simulink library "Robot_daVinci_Lib"  (R2025b)
settings: Solver=VariableStepAuto  StartTime=0.0  StopTime=10.0  RelTol=1e-3
settings Model: Creator=raissare  LastModifiedBy=guilhermepifferchristo
settings RTWCC: GPUComputeCapability=3.5

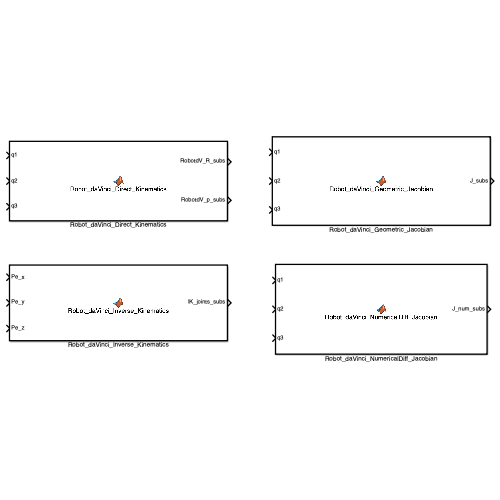
[thumbnail: Simulink's stored preview of the top-level diagram]
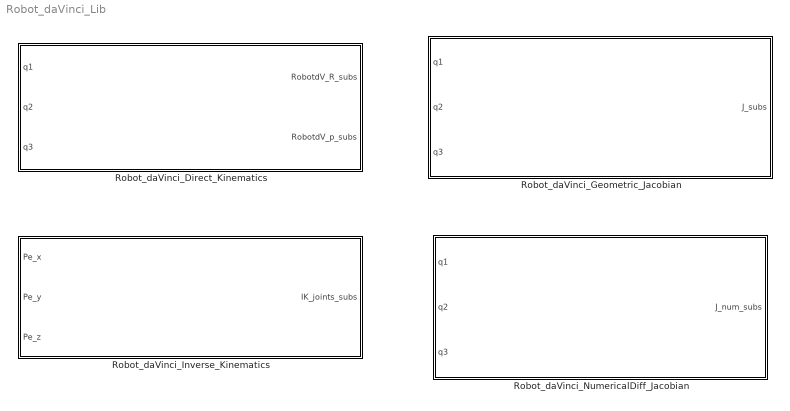
== system Robot_daVinci_Lib ==
  Robot_daVinci_Direct_Kinematics : MATLAB Function  TreatAsAtomicUnit=on
  Robot_daVinci_Geometric_Jacobian : MATLAB Function  TreatAsAtomicUnit=on
  Robot_daVinci_Inverse_Kinematics : MATLAB Function  TreatAsAtomicUnit=on
  Robot_daVinci_NumericalDiff_Jacobian : MATLAB Function  TreatAsAtomicUnit=on

== matlab function Robot_daVinci_Lib/Robot_daVinci_Geometric_Jacobian ==
  data: q1 input; J_subs output; q2 input; q3 input
function J_subs = Robot_daVinci_Geometric_Jacobian(q1,q2,q3)
%#codegen

%    This function was generated by the Symbolic Math Toolbox version 25.2.
%    10-May-2026 17:21:34

% q1 = complex(q1);  % if required to enforce complex operations
% q2 = complex(q2);  % if required to enforce complex operations
% q3 = complex(q3);  % if required to enforce complex operations
t2 = cos(q1);
t3 = cos(q2);
t4 = sin(q1);
t5 = sin(q2);
t6 = q3.*t3;
t7 = q3.*t2.*t5;
t8 = q3.*t4.*t5;
t10 = t5./1.0e+1;
t11 = (t2.*t3)./1.0e+1;
t12 = (t3.*t4)./1.0e+1;
t9 = -t6;
t14 = t7+t11;
t13 = t9+t10;
J_subs = reshape([-t8-t12,t14,0.0,0.0,0.0,1.0,-t2.*t13,-t4.*t13,t4.*(t8+t12)+t2.*t14,t4,-t2,0.0,t2.*t5,t4.*t5,-t3,0.0,0.0,0.0],[6,3]);
end

== matlab function Robot_daVinci_Lib/Robot_daVinci_Direct_Kinematics ==
  data: q1 input; RobotdV_R_subs output; q2 input; q3 input; RobotdV_p_subs output
function [RobotdV_R_subs,RobotdV_p_subs] = Robot_daVinci_Direct_Kinematics(q1,q2,q3)
%#codegen

%    This function was generated by the Symbolic Math Toolbox version 25.2.
%    10-May-2026 17:21:32

% q1 = complex(q1);  % if required to enforce complex operations
% q2 = complex(q2);  % if required to enforce complex operations
% q3 = complex(q3);  % if required to enforce complex operations
t2 = cos(q1);
t3 = cos(q2);
t4 = sin(q1);
t5 = sin(q2);
RobotdV_R_subs = reshape([t2.*t3,t3.*t4,t5,t4,-t2,0.0,t2.*t5,t4.*t5,-t3],[3,3]);
if nargout > 1
    t6 = q3.*t5;
    t7 = t3./1.0e+1;
    t8 = t6+t7;
    RobotdV_p_subs = [t2.*t8;t4.*t8;t5./1.0e+1-q3.*t3];
end
end

== matlab function Robot_daVinci_Lib/Robot_daVinci_NumericalDiff_Jacobian ==
  data: q1 input; J_num_subs output; q2 input; q3 input
function J_num_subs = Robot_daVinci_NumericalDiff_Jacobian(q1,q2,q3)
%#codegen

%    This function was generated by the Symbolic Math Toolbox version 25.2.
%    10-May-2026 17:21:34

% q1 = complex(q1);  % if required to enforce complex operations
% q2 = complex(q2);  % if required to enforce complex operations
% q3 = complex(q3);  % if required to enforce complex operations
t2 = cos(q1);
t3 = cos(q2);
t4 = sin(q1);
t5 = sin(q2);
t10 = q1+1.0e-6;
t11 = q2+1.0e-6;
t6 = t3.^2;
t7 = t5.^2;
t8 = q3.*t5;
t9 = t3./1.0e+1;
t12 = t2.*t4.*1.0e+6;
t13 = cos(t10);
t14 = cos(t11);
t15 = sin(t10);
t16 = sin(t11);
t20 = t3.*1.00001e-1;
t17 = t8+t9;
t18 = -t12;
t19 = q3.*t16;
t21 = t14./1.0e+1;
t22 = t8+t20;
t23 = t2.*t17.*1.0e+6;
t24 = t4.*t17.*1.0e+6;
t27 = t19+t21;
t25 = -t23;
t26 = -t24;
mt1 = [t25+t2.*t22.*1.0e+6,t26+t4.*t22.*1.0e+6,t5,0.0,0.0,t18+t6.*t12+t7.*t12,t25+t13.*t17.*1.0e+6,t26+t15.*t17.*1.0e+6,0.0,0.0,0.0,t4.*t13.*-1.0e+6+t2.*t6.*t15.*1.0e+6+t2.*t7.*t15.*1.0e+6,t25+t2.*t27.*1.0e+6,t26+t4.*t27.*1.0e+6,t5.*-1.0e+5+t16.*1.0e+5+q3.*t3.*1.0e+6-q3.*t14.*1.0e+6,t3.*t4.*t16.*1.0e+6-t4.*t5.*t14.*1.0e+6];
mt2 = [t2.*t3.*t16.*-1.0e+6+t2.*t5.*t14.*1.0e+6,t18+t3.*t12.*t14+t5.*t12.*t16];
J_num_subs = reshape([mt1,mt2],6,3);
end

== matlab function Robot_daVinci_Lib/Robot_daVinci_Inverse_Kinematics ==
  data: Pe_x input; IK_joints_subs output; Pe_y input; Pe_z input
function IK_joints_subs = Robot_daVinci_Inverse_Kinematics(Pe_x,Pe_y,Pe_z)
%#codegen

%    This function was generated by the Symbolic Math Toolbox version 25.2.
%    10-May-2026 17:21:33

% Pe_x = complex(Pe_x);  % if required to enforce complex operations
% Pe_y = complex(Pe_y);  % if required to enforce complex operations
% Pe_z = complex(Pe_z);  % if required to enforce complex operations
t2 = Pe_x.^2;
t3 = Pe_y.^2;
t4 = Pe_z.^2;
t5 = Pe_y.*1i;
t6 = Pe_z.*1i;
t7 = Pe_x+t5;
t8 = t2+t3;
t9 = angle(t7);
t10 = sqrt(t8);
t11 = t4+t8-1.0./1.0e+2;
t12 = t6+t10;
t14 = sqrt(t11);
t13 = angle(t12);
t15 = t14.*1i;
t16 = t15+1.0./1.0e+1;
t17 = angle(t16);
IK_joints_subs = reshape([t9,t9,t13+t17,t13-t17,t14,-t14],[2,3]);
end
